simulink model "lab2"  (R2023a)
settings: Solver=FixedStepAuto  StartTime=0.0  StopTime=20  FixedStep=0.001  RelTol=1e-3
settings Model: Creator=alaam  LastModifiedBy=alaam

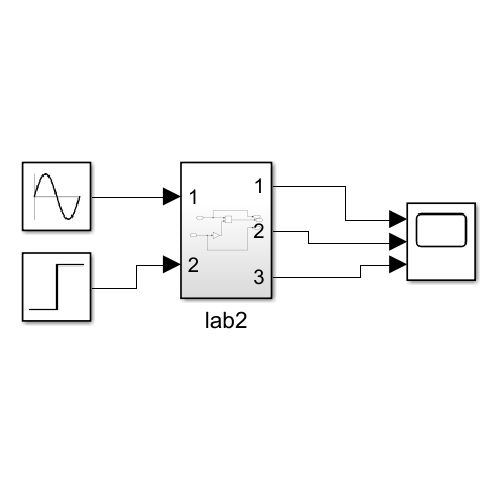
[thumbnail: Simulink's stored preview of the top-level diagram]
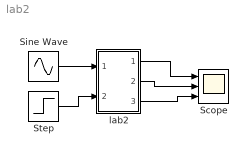
== system lab2 ==
  Scope : Scope  NumInputPorts=3
  Sine Wave : Sin  Phase=2*pi*1  SampleTime=0
  Step : Step  Time=2  SampleTime=0
  lab2 : Subsystem
  wires:
  lab2/1(Out1) -> Scope/1
  lab2/2(Out2) -> Scope/2
  lab2/3(Out3) -> Scope/3
  Sine Wave/1 -> lab2/1(Input)
  Step/1 -> lab2/2(Input1)

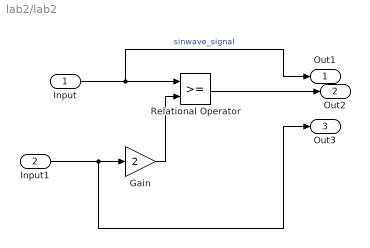
== system lab2/lab2 ==
  Input : Inport
  Input1 : Inport  Port=2
  Gain : Gain  Gain=2
  Relational Operator : RelationalOperator  OutDataTypeStr=boolean  RndMeth=Simplest  InputSameDT=off
  Out1 : Outport
  Out2 : Outport  Port=2
  Out3 : Outport  Port=3
  wires:
  Input/1 -> Out1/1, Relational Operator/1  "sinwave_signal"
  Relational Operator/1 -> Out2/1
  Input1/1 -> Out3/1, Gain/1
  Gain/1 -> Relational Operator/2
